simulink model "CLLLC_forward"  (R2021a)
settings: Solver=VariableStepAuto  StartTime=0.0  StopTime=0.1  RelTol=1e-3
undefined symbols (not defined in the file): Lm
libraries: spsSeriesRLCBranchLib x20, spsDiodeLib x8, spsIGBTDiodeLib x8, spsVoltageMeasurementLib x4, spsCurrentMeasurementLib x2, spsDCVoltageSourceLib x2, spsMultimeterLib x2, spsRMSLib x2, spsLinearTransformerLib x1, spspowerguiLib x1
settings Model: Creator=sy167  LastModifiedBy=zhang
settings SolverCC: AlgebraicLoopSolver=TrustRegion
settings DataIOCC: ReturnWorkspaceOutputs=off
settings DebuggingCC: SFMachineParentedDataDiag=warning  ArithmeticOperatorsInVariantConditions=warning
settings SFSimCC: SimUseLocalCustomCode=off  CustomCodeUndefinedFunction=UseInterfaceOnly
settings RTWCC: RTWUseLocalCustomCode=off

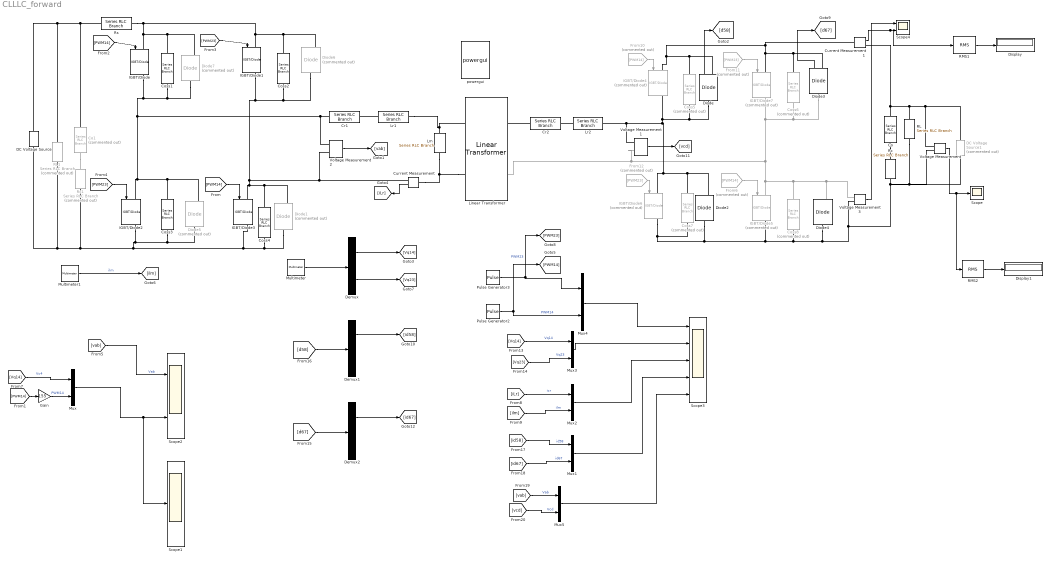
== system CLLLC_forward ==
  Co : spsSeriesRLCBranchLib/Series RLC Branch  LConnTagsString=__new0  RConnTagsString=__new0  BranchType=C  Resistance=1  Inductance=72e-6  SetiL0=off  InitialCurrent=0  Capacitance=2200e-6  Setx0=off  InitialVoltage=1500  Measurements=Branch voltage
  Co1 : spsSeriesRLCBranchLib/Series RLC Branch  Commented=on  LConnTagsString=__new0  RConnTagsString=__new0  BranchType=C  Resistance=1  Inductance=72e-6  SetiL0=off  InitialCurrent=0  Capacitance=2200e-6  Setx0=off  InitialVoltage=1500  Measurements=Branch voltage
  Coss1 : spsSeriesRLCBranchLib/Series RLC Branch  LConnTagsString=__new0  RConnTagsString=__new0  BranchType=C  Resistance=1  Inductance=72e-6  SetiL0=off  InitialCurrent=0  Capacitance=1000e-12  Setx0=off  InitialVoltage=0  Measurements=Branch voltage
  Coss2 : spsSeriesRLCBranchLib/Series RLC Branch  LConnTagsString=__new0  RConnTagsString=__new0  BranchType=C  Resistance=1  Inductance=72e-6  SetiL0=off  InitialCurrent=0  Capacitance=1000e-12  Setx0=off  InitialVoltage=0  Measurements=Branch voltage
  Coss3 : spsSeriesRLCBranchLib/Series RLC Branch  LConnTagsString=__new0  RConnTagsString=__new0  BranchType=C  Resistance=1  Inductance=72e-6  SetiL0=off  InitialCurrent=0  Capacitance=1000e-12  Setx0=off  InitialVoltage=0  Measurements=None
  Coss4 : spsSeriesRLCBranchLib/Series RLC Branch  LConnTagsString=__new0  RConnTagsString=__new0  BranchType=C  Resistance=1  Inductance=72e-6  SetiL0=off  InitialCurrent=0  Capacitance=1000e-12  Setx0=off  InitialVoltage=0  Measurements=Branch current
  Coss5 : spsSeriesRLCBranchLib/Series RLC Branch  Commented=on  LConnTagsString=__new0  RConnTagsString=__new0  BranchType=C  Resistance=1  Inductance=72e-6  SetiL0=off  InitialCurrent=0  Capacitance=1000e-12  Setx0=off  InitialVoltage=0  Measurements=None
  Coss6 : spsSeriesRLCBranchLib/Series RLC Branch  Commented=on  LConnTagsString=__new0  RConnTagsString=__new0  BranchType=C  Resistance=1  Inductance=72e-6  SetiL0=off  InitialCurrent=0  Capacitance=1000e-12  Setx0=off  InitialVoltage=0  Measurements=None
  Coss7 : spsSeriesRLCBranchLib/Series RLC Branch  Commented=on  LConnTagsString=__new0  RConnTagsString=__new0  BranchType=C  Resistance=1  Inductance=72e-6  SetiL0=off  InitialCurrent=0  Capacitance=1000e-12  Setx0=off  InitialVoltage=0  Measurements=None
  Coss8 : spsSeriesRLCBranchLib/Series RLC Branch  Commented=on  LConnTagsString=__new0  RConnTagsString=__new0  BranchType=C  Resistance=1  Inductance=72e-6  SetiL0=off  InitialCurrent=0  Capacitance=1000e-12  Setx0=off  InitialVoltage=0  Measurements=Branch current
  Cr1 : spsSeriesRLCBranchLib/Series RLC Branch  LConnTagsString=__new0  RConnTagsString=__new0  BranchType=C  Resistance=1  Inductance=72e-6  SetiL0=off  InitialCurrent=0  Capacitance=31.22e-9  Setx0=off  InitialVoltage=0  Measurements=None
  Cr2 : spsSeriesRLCBranchLib/Series RLC Branch  LConnTagsString=__new0  RConnTagsString=__new0  BranchType=C  Resistance=1  Inductance=72e-6  SetiL0=off  InitialCurrent=0  Capacitance=1.13e-6  Setx0=off  InitialVoltage=0  Measurements=Branch current
  Current Measurement : spsCurrentMeasurementLib/Current Measurement  PhasorSimulation=off  OutputType=Complex  PSBequivalent=0
  Current Measurement1 : spsCurrentMeasurementLib/Current Measurement  PhasorSimulation=off  OutputType=Complex  PSBequivalent=0
  DC Voltage Source : spsDCVoltageSourceLib/DC Voltage Source  Amplitude=700  Measurements=None
  DC Voltage Source1 : spsDCVoltageSourceLib/DC Voltage Source  Commented=on  Amplitude=311  Measurements=None
  Demux : Demux  Outputs=2
  Demux1 : Demux  Outputs=2
  Demux2 : Demux  Outputs=2
  Diode{,2..4} (4 alike) : spsDiodeLib/Diode  Ron=0.001  Lon=0  Vf=0.8  IC=0  UseSnubber=0  Rs=500  Cs=250e-9  Measurements=on
  Diode{1,5..7} (4 alike) : spsDiodeLib/Diode  Commented=on  Ron=0.001  Lon=0  Vf=0.8  IC=0  UseSnubber=0  Rs=500  Cs=250e-9  Measurements=on
  Display : Display
  Display1 : Display
  From10 : From  Commented=on  GotoTag=PWM14
  From11 : From  Commented=on  GotoTag=PWM23
  From12 : From  Commented=on  GotoTag=PWM23
  From6 : From  Commented=on  GotoTag=PWM14
  Gain : Gain  Gain=155
  IGBT/Diode{,1..3} (4 alike) : spsIGBTDiodeLib/IGBT//Diode  Ron=1e-3  Rs=1e5  Cs=inf  Measurements=on
  IGBT/Diode{4..7} (4 alike) : spsIGBTDiodeLib/IGBT//Diode  Commented=on  Ron=1e-3  Rs=1e5  Cs=inf  Measurements=on
  Linear Transformer : spsLinearTransformerLib/Linear Transformer  UNITS=SI  NominalPower=[ 250e6 100e3]  winding1=[6.5 0 0]  winding2=[1 0 0]  ThreeWindings=off  winding3=[1 0 0]  RmLm=[1e6 inf]  Measurements=None  DataType=on
  Lm : spsSeriesRLCBranchLib/Series RLC Branch  LConnTagsString=__new0  RConnTagsString=__new0  BranchType=L  Resistance=1  Inductance=202.82e-6  SetiL0=off  InitialCurrent=0  Capacitance=1e-6  Setx0=off  InitialVoltage=0  Measurements=Branch current
  Lr1 : spsSeriesRLCBranchLib/Series RLC Branch  LConnTagsString=__new0  RConnTagsString=__new0  BranchType=L  Resistance=1  Inductance=81.13e-6  SetiL0=off  InitialCurrent=0  Capacitance=1e-6  Setx0=off  InitialVoltage=0  Measurements=None
  Lr2 : spsSeriesRLCBranchLib/Series RLC Branch  LConnTagsString=__new0  RConnTagsString=__new0  BranchType=L  Resistance=1  Inductance=1.93e-6  SetiL0=off  InitialCurrent=0  Capacitance=1e-6  Setx0=off  InitialVoltage=0  Measurements=None
  Multimeter : spsMultimeterLib/Multimeter  PhasorSimulation=off  OutputType=Complex  sel=[2 3]  L=7  Gain=[1 1]  yselected={'Ub: Coss1','Ub: Coss2'};  PSBOutputType=1  PSBequivalent=0  AxesSetting=[0,0.1,-100,100]  Display=0  SavedBlockNames=-11
  Multimeter1 : spsMultimeterLib/Multimeter  PhasorSimulation=off  OutputType=Complex  sel=6  L=7  Gain=1  yselected={'Ib: Lm'};  PSBOutputType=1  PSBequivalent=0  AxesSetting=[0,0.1,-100,100]  Display=0  SavedBlockNames=-11
  Mux{,1..5} (6 alike) : Mux  Inputs=2
  Pulse Generator2 : DiscretePulseGenerator  PulseType=Time based  Period=1/110e3  PulseWidth=45
  Pulse Generator3 : DiscretePulseGenerator  PulseType=Time based  Period=1/110e3  PulseWidth=45  PhaseDelay=1/110e3/2
  RL : spsSeriesRLCBranchLib/Series RLC Branch  LConnTagsString=__new0  RConnTagsString=__new0  BranchType=R  Resistance=(48*48)/1000  Inductance=Lm  SetiL0=off  InitialCurrent=0  Capacitance=1e-6  Setx0=off  InitialVoltage=0  Measurements=None
  RL1 : spsSeriesRLCBranchLib/Series RLC Branch  Commented=on  LConnTagsString=__new0  RConnTagsString=__new0  BranchType=R  Resistance=48/(20)  Inductance=Lm  SetiL0=off  InitialCurrent=0  Capacitance=1e-6  Setx0=off  InitialVoltage=0  Measurements=None
  RMS1 : spsRMSLib/RMS  TrueRMS=on  Freq=100e3  RMSInit=120  Ts=0
  RMS2 : spsRMSLib/RMS  TrueRMS=on  Freq=100e3  RMSInit=120  Ts=0
  Rc : spsSeriesRLCBranchLib/Series RLC Branch  LConnTagsString=__new0  RConnTagsString=__new0  BranchType=R  Resistance=5e-3  Inductance=Lm  SetiL0=off  InitialCurrent=0  Capacitance=1e-6  Setx0=off  InitialVoltage=0  Measurements=None
  Rc1 : spsSeriesRLCBranchLib/Series RLC Branch  Commented=on  LConnTagsString=__new0  RConnTagsString=__new0  BranchType=R  Resistance=5e-3  Inductance=Lm  SetiL0=off  InitialCurrent=0  Capacitance=1e-6  Setx0=off  InitialVoltage=0  Measurements=None
  Rs : spsSeriesRLCBranchLib/Series RLC Branch  LConnTagsString=__new0  RConnTagsString=__new0  BranchType=R  Resistance=1e-6  Inductance=6.45e-6  SetiL0=off  InitialCurrent=0  Capacitance=1e-6  Setx0=off  InitialVoltage=0  Measurements=Branch current
  Scope : Scope
  Scope1 : Scope
  Scope2 : Scope  NumInputPorts=2
  Scope3 : Scope  NumInputPorts=5
  Scope4 : Scope  NumInputPorts=2
  Voltage Measurement{,1..3} (4 alike) : spsVoltageMeasurementLib/Voltage Measurement  PhasorSimulation=off  OutputType=Complex  PSBequivalent=0
  powergui : spspowerguiLib/powergui  Priority=1  SimulationMode=Discrete  SampleTime=1/200e3/100  frequency=60  Iterations=50  frequencyindice=0  Pbase=100e6  ErrMax=1e-4  UnitsV=kV  UnitsW=MW  buscounter=0  FunctionMessages=off  echomessages=off  EnableUseOfTLC=off  CurrentSourceSwitches=off  DisableSnubberDevices=off  DisableRonSwitches=off  DisableVfSwitches=off  DisplayEquations=off  AutomaticDiscreteSolvers=off  SolverType=Tustin/Backward Euler (TBE)  Interpol=off  ExternalGateDelay=off  methode=off  Ts=100  x0status=blocks  SPID=off  SwTol=0  HookPort=off  NonlinearTolerance=1e-4  nMaxIteration=100  ContinueOnMaxIteration=off  RestoreLinks=warning  ResistiveCurrentMeasurement=off  Frange=[0:2:500]  Ylog=off  Xlog=on  ShowGrid=off  save=off  variable=ZData  structure=0  ZoomFFT=on  StartTime=0.0  cycles=1  DisplayStyle=1  fundamental=60  FreqAxis=off  MaxFrequency=1000  frequencyindicesteady=1  RmsSteady=1  display=off
  wires:
  [PWM14] -> Gain/1
  [PWM14] -> IGBT/Diode/1
  Voltage Measurement2/1 -> [vab]
  [Vq14] -> Mux/1  "Vc4"
  [vab] -> Scope2/1  "Vab"
  Gain/1 -> Mux/2  "PWM14"
  Mux/1 -> Scope1/1, Scope2/2
  [PWM23] -> IGBT/Diode1/1
  [PWM14] -> IGBT/Diode3/1
  Current Measurement/1 -> [iLr]
  [PWM23] -> IGBT/Diode2/1
  Current Measurement1/1 -> RMS1/1, Scope4/2
  From11/1 -> IGBT/Diode7/1
  From12/1 -> IGBT/Diode6/1
  From6/1 -> IGBT/Diode5/1
  Voltage Measurement3/1 -> Scope4/1
  From10/1 -> IGBT/Diode4/1
  [iLr] -> Mux2/1  "icr"
  Multimeter1/1 -> [ilm]  "ilm"
  [ilm] -> Mux2/2  "ilm"
  Multimeter/1 -> Demux/1
  Demux/1 -> [Vq14]
  Demux/2 -> [Vq23]
  [Vq14] -> Mux3/1  "Vq14"
  [Vq23] -> Mux3/2  "Vq23"
  Mux3/1 -> Scope3/2
  Mux4/1 -> Scope3/1
  Pulse Generator3/1 -> Mux4/1, [PWM23]  "PWM23"
  Pulse Generator2/1 -> [PWM14], Mux4/2  "PWM14"
  Mux2/1 -> Scope3/3
  Diode/1 -> [d58]
  Diode3/1 -> [d67]
  Demux1/1 -> [id58]
  Demux2/1 -> [id67]
  [d58] -> Demux1/1
  [d67] -> Demux2/1
  Mux1/1 -> Scope3/4
  [id58] -> Mux1/1  "id58"
  [id67] -> Mux1/2  "id67"
  RMS1/1 -> Display/1
  Voltage Measurement/1 -> RMS2/1, Scope/1
  RMS2/1 -> Display1/1
  Mux5/1 -> Scope3/5
  [vcd] -> Mux5/2  "Vcd"
  [vab] -> Mux5/1  "Vab"
  Voltage Measurement1/1 -> [vcd]
  connections:
  Linear Transformer/LConn1 -- Lm/LConn1 -- Lr1/RConn1
  Coss4/RConn1 -- Diode1/LConn1 -- IGBT/Diode3/RConn1 -- Diode5/LConn1 -- Coss3/RConn1 -- IGBT/Diode2/RConn1 -- RL1/RConn1 -- DC Voltage Source/LConn1 -- Rc1/RConn1
  Coss1/LConn1 -- Diode7/RConn1 -- IGBT/Diode/LConn1 -- Diode6/RConn1 -- Coss2/LConn1 -- IGBT/Diode1/LConn1 -- Rs/RConn1
  Coss4/LConn1 -- Diode1/RConn1 -- IGBT/Diode3/LConn1 -- Diode6/LConn1 -- Coss2/RConn1 -- IGBT/Diode1/RConn1 -- Voltage Measurement2/LConn2 -- Current Measurement/RConn1
  Coss3/LConn1 -- Diode5/RConn1 -- IGBT/Diode2/LConn1 -- Diode7/LConn1 -- Coss1/RConn1 -- IGBT/Diode/RConn1 -- Cr1/LConn1 -- Voltage Measurement2/LConn1
  Linear Transformer/LConn2 -- Lm/RConn1 -- Current Measurement/LConn1
  Co/RConn1 -- Rc/LConn1
  Lr1/LConn1 -- Cr1/RConn1
  DC Voltage Source/RConn1 -- Co1/LConn1 -- Rs/LConn1 -- RL1/LConn1
  IGBT/Diode4/LConn1 -- Diode/RConn1 -- Coss5/LConn1 -- Current Measurement1/LConn1 -- Diode3/RConn1 -- Coss6/LConn1 -- IGBT/Diode7/LConn1
  Co/LConn1 -- Current Measurement1/RConn1 -- DC Voltage Source1/RConn1 -- Voltage Measurement/LConn1 -- RL/LConn1
  Coss8/LConn1 -- Diode4/RConn1 -- Voltage Measurement3/LConn1 -- IGBT/Diode5/LConn1 -- Voltage Measurement1/LConn2 -- Linear Transformer/RConn2 -- Diode3/LConn1 -- Coss6/RConn1 -- IGBT/Diode7/RConn1
  IGBT/Diode5/RConn1 -- Diode2/LConn1 -- IGBT/Diode6/RConn1 -- Coss7/RConn1 -- Coss8/RConn1 -- Rc/RConn1 -- RL/RConn1 -- Voltage Measurement/LConn2 -- DC Voltage Source1/LConn1 -- Voltage Measurement3/LConn2 -- Diode4/LConn1
  Co1/RConn1 -- Rc1/LConn1
  Lr2/LConn1 -- Cr2/RConn1
  Cr2/LConn1 -- Linear Transformer/RConn1
  Diode/LConn1 -- Coss5/RConn1 -- Voltage Measurement1/LConn1 -- Lr2/RConn1 -- Diode2/RConn1 -- Coss7/LConn1 -- IGBT/Diode6/LConn1 -- IGBT/Diode4/RConn1
